simulink model "rlwatertank_3"  (R2023b)
settings: Solver=ode45  StartTime=0.0  StopTime=inf  RelTol=1e-3  EnableMultiTasking=on
undefined symbols (not defined in the file): DiscIntNeverNeededParam, Ts
libraries: simulink x4, rllib x1
settings Model: Creator=The MathWorks, Inc.  LastModifiedBy=hdt
settings SolverCC: AlgebraicLoopSolver=TrustRegion
settings DataIOCC: LimitDataPoints=on  SaveFormat=Array  SignalLoggingName=logsOut
settings OptimizationCC: ExpressionDepthLimit=2147483647  InitFltsAndDblsToZero=on  LifeSpan=inf
settings DebuggingCC: SaveWithParameterizedLinksMsg=none  UnderspecifiedInitializationDetection=Classic  MergeDetectMultiDrivingBlocksExec=none  SignalResolutionControl=TryResolveAllWithWarning  MultiTaskDSMMsg=warning  FcnCallInpInsideContextMsg=warning  UnconnectedInputMsg=warning  UnconnectedOutputMsg=warning  UnconnectedLineMsg=warning  AllowSymbolicDim=off  StateNameClashWarn=warning  SFUnexpectedBacktrackingDiag=warning  SFNoUnconditionalDefaultTransitionDiag=warning  SFExecutionAtInitializationDiag=none  ArithmeticOperatorsInVariantConditions=warning
settings HardwareCC: ProdBitPerPointer=32  ProdBitPerSizeT=32  ProdBitPerPtrDiffT=32  ProdLargestAtomicFloat=None  ProdIntDivRoundTo=Undefined  ProdEndianess=Unspecified  ProdWordSize=32  ProdHWDeviceType=Specified
settings ModelReferenceCC: EnableRefExpFcnMdlSchedulingChecks=on  PropagateSignalLabelsOutOfModel=off
settings SFSimCC: SimUseLocalCustomCode=off
settings RTWCC: RTWUseLocalCustomCode=off
settings CodeAppCC: StateflowObjectComments=on
settings GRTTargetCC: TargetFcnLib=ansi_tfl_tmw.mat  TargetLangStandard=C89/C90 (ANSI)  CombineOutputUpdateFcns=off  GRTInterface=on
settings ConfigComp: CovMetricSettings=dw  CovSaveCumulativeToWorkspaceVar=on  CovSaveSingleToWorkspaceVar=on  CovExternalEMLEnable=off

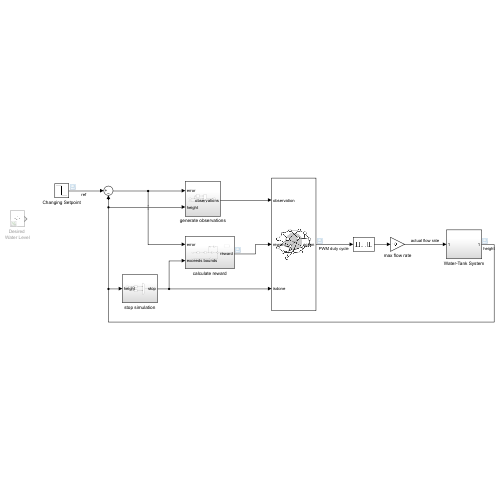
[thumbnail: Simulink's stored preview of the top-level diagram]
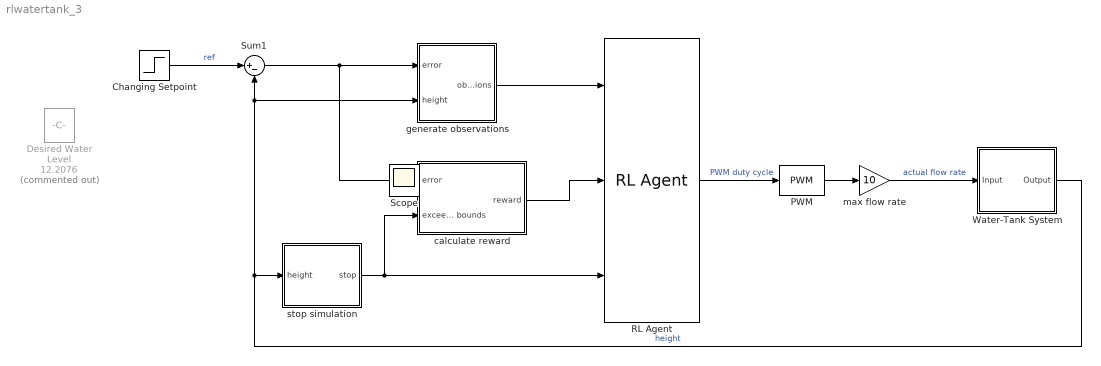
== system rlwatertank_3 ==
  Changing Setpoint : Step  Time=101  Before=16.7324  After=12.2239  SampleTime=0
  Desired Water Level : Constant  Commented=on  Value=12.2076
  PWM : simulink/Discontinuities/PWM  DisableCoverage=on  Period=0.1  InitialDelay=0  DisallowZeroDutyCycle=off  RunAtFixedTimeIntervals=off  SampleTime=0.1
  RL Agent : rllib/RL Agent  Agent=agent_Trained_1  ExternalActionAsInput=off  ProvideLastAction=off  ProvideCumRwd=off  TreatAsDirectFeedthrough=on  UseStrictObservationDataTypes=off
  Sum1 : Sum  Inputs=|+-  SaturateOnIntegerOverflow=on
  Water-Tank System : Subsystem
  calculate reward : Subsystem
  generate observations : Subsystem
  max flow rate : Gain  Gain=10
  stop simulation : Subsystem
  Scope : Scope
  wires:
  Changing Setpoint/1 -> Sum1/1  "ref"
  Sum1/1 -> calculate reward/1(error), generate observations/1(error)
  Water-Tank System/1(Output) -> stop simulation/1(height), Sum1/2, generate observations/2(height)  "height"
  RL Agent/1 -> PWM/1  "PWM duty cycle"
  stop simulation/1(stop) -> calculate reward/2(exceeds bounds), RL Agent/3
  generate observations/1(observations) -> RL Agent/1
  calculate reward/1(reward) -> RL Agent/2
  PWM/1 -> max flow rate/1
  max flow rate/1 -> Water-Tank System/1(Input)  "actual flow rate"

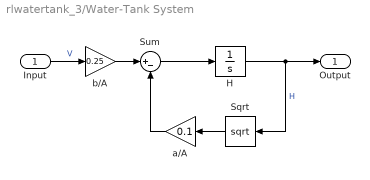
== system rlwatertank_3/Water-Tank System ==
  Input : Inport
  H : Integrator  InitialCondition=10.235  LimitOutput=on  LowerSaturationLimit=0
  Sqrt : Sqrt  OutputSignalType=real
  Sum : Sum  Inputs=|+-  SaturateOnIntegerOverflow=on
  a/A : Gain  Gain=0.1  SaturateOnIntegerOverflow=on  OutDataTypeStr=Inherit: Same as input  ParamDataTypeStr=Inherit: Same as input
  b/A : Gain  Gain=0.25  SaturateOnIntegerOverflow=on  OutDataTypeStr=Inherit: Same as input  ParamDataTypeStr=Inherit: Same as input
  Output : Outport  VectorParamsAs1DForOutWhenUnconnected=off
  wires:
  b/A/1 -> Sum/1
  Sum/1 -> H/1
  H/1 -> Sqrt/1, Output/1  "H"
  Sqrt/1 -> a/A/1
  a/A/1 -> Sum/2
  Input/1 -> b/A/1  "V"

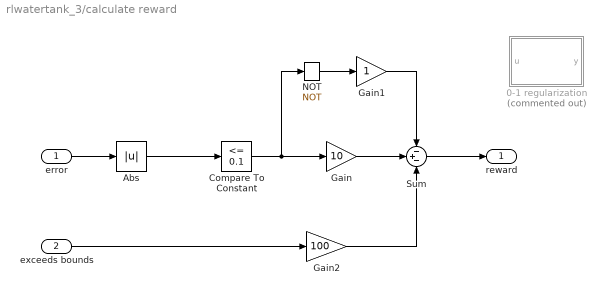
== system rlwatertank_3/calculate reward ==
  error : Inport
  exceeds bounds : Inport  Port=2
  0-1 regularization : MATLAB Function  Commented=on  TreatAsAtomicUnit=on
  Abs : Abs  SaturateOnIntegerOverflow=off
  Compare To Constant : simulink/Logic and Bit Operations/Compare To Constant  relop=<=  const=0.1  OutDataTypeStr=boolean
  Gain : Gain  Gain=10
  Gain1 : Gain
  Gain2 : Gain  Gain=100
  NOT : Logic  Operator=NOT  IconShape=distinctive  AllPortsSameDT=off  OutDataTypeStr=boolean
  Sum : Sum  Inputs=-+-  OutDataTypeStr=double
  reward : Outport  VectorParamsAs1DForOutWhenUnconnected=off
  wires:
  Abs/1 -> Compare To Constant/1
  Gain2/1 -> Sum/3
  exceeds bounds/1 -> Gain2/1
  error/1 -> Abs/1
  Gain/1 -> Sum/2
  Sum/1 -> reward/1
  Compare To Constant/1 -> NOT/1, Gain/1
  Gain1/1 -> Sum/1
  NOT/1 -> Gain1/1

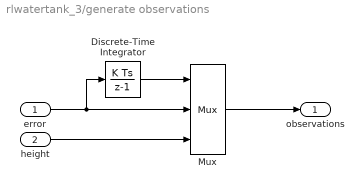
== system rlwatertank_3/generate observations ==
  error : Inport
  height : Inport  Port=2
  Discrete-Time Integrator : DiscreteIntegrator  SampleTime=Ts  ICPrevOutput=DiscIntNeverNeededParam  ICPrevScaledInput=DiscIntNeverNeededParam
  Mux : Mux  Inputs=3
  observations : Outport  VectorParamsAs1DForOutWhenUnconnected=off
  wires:
  height/1 -> Mux/3
  Discrete-Time Integrator/1 -> Mux/1
  error/1 -> Mux/2, Discrete-Time Integrator/1
  Mux/1 -> observations/1

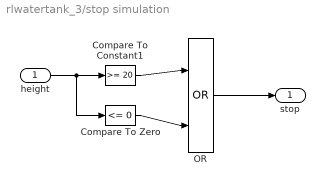
== system rlwatertank_3/stop simulation ==
  height : Inport
  Compare To Constant1 : simulink/Logic and Bit Operations/Compare To Constant  relop=>=  const=20  OutDataTypeStr=boolean
  Compare To Zero : simulink/Logic and Bit Operations/Compare To Zero  relop=<=  OutDataTypeStr=boolean
  OR : Logic  Operator=OR  IconShape=distinctive  AllPortsSameDT=off  OutDataTypeStr=boolean
  stop : Outport  VectorParamsAs1DForOutWhenUnconnected=off
  wires:
  height/1 -> Compare To Zero/1, Compare To Constant1/1
  Compare To Zero/1 -> OR/2
  Compare To Constant1/1 -> OR/1
  OR/1 -> stop/1

== matlab function rlwatertank_3/calculate reward/0-1 regularization ==
  data: u input; y output
function y = fcn(u)
    min = -200;
    max = 2000;
    y = (u-min)/(max-min);
end
